simulink library "suspention"  (R2019b)
settings: Solver=ode45  StartTime=0.0  StopTime=10.0  RelTol=1e-3
PostLoadFcn:
  | setsysloc libsb2slobsolete
undefined symbols (not defined in the file): A, Ac, Ad, B, Bc, Bd, C, Cc, Cd, code, const, D, data, Dc, Dd, DiscIntNeverNeededParam, gain, info, k, m, map, no, stat, X0, xd, xi
libraries: $bdroot x2, simulink x2, libsb2sl x1
(part 2 of 2)

== system suspention/DYN/DResetIntegrator ==
  1stOrder : Subsystem  mask(DYN-Palette){IMODE=Forward Euler, RMODE=Single edge, K=1, X0=0, TS=0.1}
      mask prompts: IMODE "Integrator Method:"; RMODE "External Reset:"; K "Output Gains:"; X0 "Initial Conditions:"; TS "Sampling Time:"
      mask help: Nth order integration of an input with resettable states.
      mask init:
      | operator={'rising','either'};
      | method={'ForwardEuler';'BackwardEuler';'Trapezoidal'};
      | set_param([gcb  '/Integrator'],'ExternalReset',operator{RMODE},'IntegratorMethod',method{IMODE});
      | [x,y]=sblibico('1stOrderReset','disc');
      mask TypeOptions IMODE: Forward Euler | Backward Euler | Trapezoidal
      mask TypeOptions RMODE: Single edge | Double edge
      mask Display: plot(0,0,1,1,x,y)
  1stOrder1 : Subsystem  mask(DYN-Palette){IMODE=Forward Euler, RMODE=Single edge, X0=0, TS=0.1}
      mask prompts: IMODE "Integrator Method:"; RMODE "External Reset:"; X0 "Initial Conditions:"; TS "Sampling Time:"
      mask help: Nth order integration of an input with resettable states.
      mask init:
      | operator={'rising','either'};
      | method={'ForwardEuler';'BackwardEuler';'Trapezoidal'};
      | set_param([gcb  '/Integrator'],'ExternalReset',operator{RMODE},'IntegratorMethod',method{IMODE});
      | [x,y]=sblibico('1stOrder1Reset','disc');
      mask TypeOptions IMODE: Forward Euler | Backward Euler | Trapezoidal
      mask TypeOptions RMODE: Single edge | Double edge
      mask Display: plot(0,0,1,1,x,y)
  NthOrder : Subsystem  mask(DYN-Palette){IMODE=Forward Euler, N=1, RMODE=Single edge, NR=1, K=1, X0=0, TS=0.1}
      mask prompts: IMODE "Integrator Method:"; N "Order of Integration:"; RMODE "External Reset:"; NR "Highest Order of Resettable State:"; K "Output Gains:"; X0 "Initial Conditions:"; TS "Sampling Time:"
      mask help: Nth order integration of an input with resettable states.
      mask init:
      | no=length(K);
      | [stateMap,resetMap]=sblibdrv('Integrator',N,no,NR);
      | operator={'rising','either'};
      | method={'ForwardEuler';'BackwardEuler';'Trapezoidal'};
      | set_param([gcb  '/Integrator'],'ExternalReset',operator{RMODE},'IntegratorMethod',method{IMODE});
      | [x,y]=sblibico('nthOrderReset','disc');
      mask TypeOptions IMODE: Forward Euler | Backward Euler | Trapezoidal
      mask TypeOptions RMODE: Single edge | Double edge
      mask Display: plot(0,0,1,1,x,y)
  NthOrder1 : Subsystem  mask(DYN-Palette){IMODE=Forward Euler, N=1, RMODE=Single edge, NR=1, X0=0, TS=0.1}
      mask prompts: IMODE "Integrator Method:"; N "Order of Integration:"; RMODE "External Reset:"; NR "Highest Order of Resettable State:"; X0 "Initial Conditions:"; TS "Sampling Time:"
      mask help: Nth order integration of an input with resettable states.
      mask init:
      | no=length(X0)/N;
      | [stateMap,resetMap]=sblibdrv('Integrator',N,no,NR);
      | operator={'rising','either'};
      | method={'ForwardEuler';'BackwardEuler';'Trapezoidal'};
      | set_param([gcb  '/Integrator'],'ExternalReset',operator{RMODE},'IntegratorMethod',method{IMODE});
      | [x,y]=sblibico('nthOrder1Reset','disc');
      mask TypeOptions IMODE: Forward Euler | Backward Euler | Trapezoidal
      mask TypeOptions RMODE: Single edge | Double edge
      mask Display: plot(0,0,1,1,x,y)

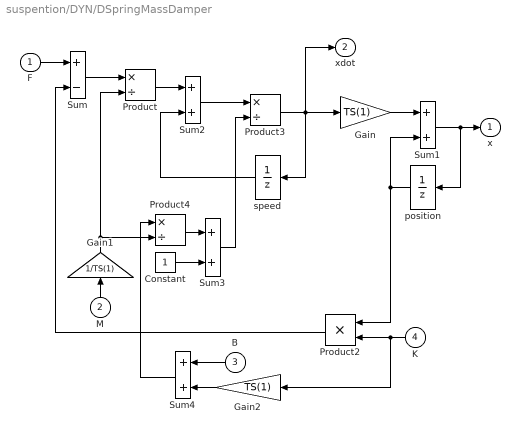
== system suspention/DYN/DSpringMassDamper ==
  F : Inport  SampleTime=TS
  M : Inport  Port=2  SampleTime=TS
  B : Inport  Port=3  SampleTime=TS
  K : Inport  Port=4  SampleTime=TS
  Constant : Constant
  Gain : Gain  Gain=TS(1)  SaturateOnIntegerOverflow=on  OutDataTypeStr=Inherit: Same as input  ParamDataTypeStr=Inherit: Same as input
  Gain1 : Gain  Gain=1/TS(1)  SaturateOnIntegerOverflow=on  OutDataTypeStr=Inherit: Same as input  ParamDataTypeStr=Inherit: Same as input
  Gain2 : Gain  Gain=TS(1)  SaturateOnIntegerOverflow=on  OutDataTypeStr=Inherit: Same as input  ParamDataTypeStr=Inherit: Same as input
  Product : Product  Inputs=*/  SaturateOnIntegerOverflow=on  RndMeth=Zero  InputSameDT=on  OutDataTypeStr=Inherit: Same as first input
  Product2 : Product  SaturateOnIntegerOverflow=on  RndMeth=Zero  InputSameDT=on  OutDataTypeStr=Inherit: Same as first input
  Product3 : Product  Inputs=*/  SaturateOnIntegerOverflow=on  RndMeth=Zero  InputSameDT=on  OutDataTypeStr=Inherit: Same as first input
  Product4 : Product  Inputs=*/  SaturateOnIntegerOverflow=on  RndMeth=Zero  InputSameDT=on  OutDataTypeStr=Inherit: Same as first input
  Sum : Sum  Inputs=+-  SaturateOnIntegerOverflow=on  InputSameDT=on  OutDataTypeStr=Inherit: Same as first input
  Sum{1..4} (4 alike) : Sum  SaturateOnIntegerOverflow=on  InputSameDT=on  OutDataTypeStr=Inherit: Same as first input
  position : UnitDelay  InitialCondition=X0(1)  SampleTime=TS  HasFrameUpgradeWarning=on
  speed : UnitDelay  InitialCondition=X0(2)  SampleTime=TS  HasFrameUpgradeWarning=on
  x : Outport  InitialOutput=X0(1)
  xdot : Outport  Port=2  InitialOutput=X0(2)
  wires:
  Sum4/1 -> Product4/1
  Gain2/1 -> Sum4/2
  B/1 -> Sum4/1
  K/1 -> Gain2/1, Product2/2
  Gain1/1 -> Product4/2, Product/2
  M/1 -> Gain1/1
  position/1 -> Product2/1, Sum1/2
  Sum3/1 -> Product3/2
  Product2/1 -> Sum/2
  Sum1/1 -> position/1, x/1
  Gain/1 -> Sum1/1
  Product3/1 -> xdot/1, Gain/1, speed/1
  Product4/1 -> Sum3/1
  Constant/1 -> Sum3/2
  speed/1 -> Sum2/2
  Sum2/1 -> Product3/1
  Product/1 -> Sum2/1
  Sum/1 -> Product/1
  F/1 -> Sum/1

== system suspention/DYN/DStateSpace ==
  u : Inport
  StateSpace : DiscreteStateSpace  A=A  B=B  C=C  D=D  InitialCondition=X0  SampleTime=TS
  y : Outport
  wires:
  u/1 -> StateSpace/1
  StateSpace/1 -> y/1

== system suspention/DYN/DTimeDelay ==
  u : Inport  SampleTime=TS
  Demux : Demux  Outputs=[no no (k+1)*no]
  Mux : Mux  Inputs=[no (k+1)*no]
  Selector : Selector  InputPortWidth=(k+2)*no  IndexOptions=Index vector (dialog)  Indices=[k*no+1:(k+2)*no 1:(k+1)*no]  OutputSizes=1
  Sum : Sum  Inputs=+|+  SaturateOnIntegerOverflow=on  InputSameDT=on  OutDataTypeStr=Inherit: Same as first input
  Unit Delay : UnitDelay  InitialCondition=X0  SampleTime=TS  HasFrameUpgradeWarning=on
  m : Gain  Gain=1-m  SaturateOnIntegerOverflow=on  OutDataTypeStr=Inherit: Same as input  ParamDataTypeStr=Inherit: Same as input
  m1 : Gain  Gain=m  SaturateOnIntegerOverflow=on  OutDataTypeStr=Inherit: Same as input  ParamDataTypeStr=Inherit: Same as input
  y : Outport
  wires:
  u/1 -> Mux/1
  Unit Delay/1 -> Mux/2
  Mux/1 -> Selector/1
  Sum/1 -> y/1
  m1/1 -> Sum/2
  m/1 -> Sum/1
  Demux/2 -> m1/1
  Demux/1 -> m/1
  Demux/3 -> Unit Delay/1
  Selector/1 -> Demux/1

== system suspention/LOG/Decoder ==
  u : Inport
  decoder : S-Function  FunctionName=sbdecoder  Parameters=BPI,MIN,MAX  SFunctionDeploymentMode=off  EnableBusSupport=off
  y : Outport
  wires:
  u/1 -> decoder/1
  decoder/1 -> y/1

== system suspention/LOG/EQV ==
  u1 : Inport
  u2 : Inport  Port=2
  EQV : Logic  Operator=NOT  Inputs=1
  NEQV : Logic  Operator=XOR
  bool1 : RelationalOperator  Operator=>  RndMeth=Nearest  InputSameDT=on
  bool2 : RelationalOperator  Operator=>  RndMeth=Nearest  InputSameDT=on
  zero : Constant  Value=0  OutDataTypeStr=Inherit: Inherit via back propagation
  y : Outport
  wires:
  bool1/1 -> NEQV/1
  bool2/1 -> NEQV/2
  u1/1 -> bool1/1
  u2/1 -> bool2/1
  zero/1 -> bool2/2, bool1/2
  NEQV/1 -> EQV/1
  EQV/1 -> y/1

== system suspention/LOG/Encoder ==
  u : Inport
  encoder : S-Function  FunctionName=sbencoder  Parameters=BPO,MIN,MAX  SFunctionDeploymentMode=off  EnableBusSupport=off
  y : Outport
  wires:
  u/1 -> encoder/1
  encoder/1 -> y/1

== system suspention/LOG/GainScheduler ==
  s : Inport
  u : Inport  Port=2
  sbgainsched : S-Function  FunctionName=sbgainsched  Parameters=IND,GAIN  SFunctionDeploymentMode=off  EnableBusSupport=off
  y : Outport
  wires:
  s/1 -> sbgainsched/1
  sbgainsched/1 -> y/1
  u/1 -> sbgainsched/2

== system suspention/LOG/LogExpression ==
  u : Inport
  sblogexp : S-Function  FunctionName=sblogexp  Parameters=code,stat,data,info,P0,TS  SFunctionDeploymentMode=off  EnableBusSupport=off
  y : Outport
  wires:
  u/1 -> sblogexp/1
  sblogexp/1 -> y/1

== system suspention/LOG/NEQV ==
  u1 : Inport
  u2 : Inport  Port=2
  NEQV : Logic  Operator=XOR
  bool1 : RelationalOperator  Operator=>  RndMeth=Nearest  InputSameDT=on
  bool2 : RelationalOperator  Operator=>  RndMeth=Nearest  InputSameDT=on
  zero : Constant  Value=0  OutDataTypeStr=Inherit: Inherit via back propagation
  y : Outport
  wires:
  bool1/1 -> NEQV/1
  bool2/1 -> NEQV/2
  u1/1 -> bool1/1
  NEQV/1 -> y/1
  u2/1 -> bool2/1
  zero/1 -> bool1/2, bool2/2

== system suspention/LOG/NOT ==
  u1 : Inport
  bool1 : RelationalOperator  Operator=>  RndMeth=Nearest  InputSameDT=on
  logic : Logic  Operator=NOT
  zero : Constant  Value=0  OutDataTypeStr=Inherit: Inherit via back propagation
  y : Outport
  wires:
  bool1/1 -> logic/1
  u1/1 -> bool1/1
  logic/1 -> y/1
  zero/1 -> bool1/2

== system suspention/LOG/ShiftRegister ==
  u : Inport  SampleTime=TS
  sbshiftreg : S-Function  FunctionName=sbshiftreg  Parameters=NX,NY,X0,TS  SFunctionDeploymentMode=off  EnableBusSupport=off
  y : Outport
  wires:
  u/1 -> sbshiftreg/1
  sbshiftreg/1 -> y/1

== system suspention/LOG/Switch ==
  u1 : Inport
  u2 : Inport  Port=2
  u3 : Inport  Port=3
  Switch : Switch  Criteria=u2 > Threshold  SaturateOnIntegerOverflow=on  InputSameDT=on
  y : Outport
  wires:
  Switch/1 -> y/1
  u2/1 -> Switch/1
  u3/1 -> Switch/3
  u1/1 -> Switch/2

== system suspention/MAT/Constant ==
  Constant : Constant  Value=constantValue
  Y : Outport
  wires:
  Constant/1 -> Y/1

== system suspention/MAT/LeftMultiply ==
  A : Inport
  Matrix Gain : Gain  Gain=G  Multiplication=Matrix(u*K)  SaturateOnIntegerOverflow=on  OutDataTypeStr=Inherit: Same as input  ParamDataTypeStr=Inherit: Same as input
  Y2y : Reshape
  a2A : Reshape  OutputDimensionality=Customize  OutputDimensions=[nACols,nARows]
  Y : Outport
  wires:
  A/1 -> a2A/1
  Y2y/1 -> Y/1
  Matrix Gain/1 -> Y2y/1
  a2A/1 -> Matrix Gain/1

== system suspention/MAT/MatLeftDivide ==
  A : Inport
  B : Inport  Port=2
  Product : Product  Inputs=*/  Multiplication=Matrix(*)  SaturateOnIntegerOverflow=on  RndMeth=Zero  InputSameDT=on  OutDataTypeStr=Inherit: Same as first input
  Y2y : Reshape
  a2A : Reshape  OutputDimensionality=Customize  OutputDimensions=[nACols,nARows]
  b2B : Reshape  OutputDimensionality=Customize  OutputDimensions=[nBCols,nBRows]
  Y : Outport
  wires:
  Product/1 -> Y2y/1
  B/1 -> b2B/1
  Y2y/1 -> Y/1
  A/1 -> a2A/1
  b2B/1 -> Product/1
  a2A/1 -> Product/2

== system suspention/MAT/MatRightDivide ==
  A : Inport
  B : Inport  Port=2
  Product : Product  Inputs=/*  Multiplication=Matrix(*)  SaturateOnIntegerOverflow=on  RndMeth=Zero  InputSameDT=on  OutDataTypeStr=Inherit: Same as first input
  Y2y : Reshape
  a2A : Reshape  OutputDimensionality=Customize  OutputDimensions=[nACols,nARows]
  b2B : Reshape  OutputDimensionality=Customize  OutputDimensions=[nBCols,nBRows]
  Y : Outport
  wires:
  b2B/1 -> Product/2
  a2A/1 -> Product/1
  Product/1 -> Y2y/1
  A/1 -> a2A/1
  Y2y/1 -> Y/1
  B/1 -> b2B/1

== system suspention/MAT/MatrixInverse ==
  A : Inport
  Product : Product  Inputs=/  Multiplication=Matrix(*)  SaturateOnIntegerOverflow=on  RndMeth=Zero  InputSameDT=on  OutDataTypeStr=Inherit: Same as first input
  Y2y : Reshape
  a2A : Reshape  OutputDimensionality=Customize  OutputDimensions=[nACols,nARows]
  Y : Outport
  wires:
  A/1 -> a2A/1
  Y2y/1 -> Y/1
  a2A/1 -> Product/1
  Product/1 -> Y2y/1

== system suspention/MAT/MatrixMultiply ==
  A : Inport
  B : Inport  Port=2
  Product : Product  Inputs=**  Multiplication=Matrix(*)  SaturateOnIntegerOverflow=on  RndMeth=Zero  InputSameDT=on  OutDataTypeStr=Inherit: Same as first input
  Y2y : Reshape
  a2A : Reshape  OutputDimensionality=Customize  OutputDimensions=[nACols,nARows]
  b2B : Reshape  OutputDimensionality=Customize  OutputDimensions=[nBCols,nBRows]
  Y : Outport
  wires:
  a2A/1 -> Product/2
  b2B/1 -> Product/1
  B/1 -> b2B/1
  Y2y/1 -> Y/1
  A/1 -> a2A/1
  Product/1 -> Y2y/1

== system suspention/MAT/MatrixTranspose ==
  A : Inport
  Selector : Selector  InputPortWidth=nARows*nACols  IndexOptions=Index vector (dialog)  Indices=mapIndices(:)  OutputSizes=1
  Y : Outport
  wires:
  Selector/1 -> Y/1
  A/1 -> Selector/1

== system suspention/MAT/RightMultiply ==
  A : Inport
  Matrix Gain : Gain  Gain=G  Multiplication=Matrix(K*u)  SaturateOnIntegerOverflow=on  OutDataTypeStr=Inherit: Same as input  ParamDataTypeStr=Inherit: Same as input
  Y2y : Reshape
  a2A : Reshape  OutputDimensionality=Customize  OutputDimensions=[nACols,nARows]
  Y : Outport
  wires:
  a2A/1 -> Matrix Gain/1
  Matrix Gain/1 -> Y2y/1
  Y2y/1 -> Y/1
  A/1 -> a2A/1

== system suspention/NTP/BiCubicInterp ==
  note: Swap inputs to accommodate
      | Row-major 2-D tables in
      | SystemBuild
  u1 : Inport
  u2 : Inport  Port=2
  Look-Up Table (n-D) : Lookup_n-D  BreakpointsForDimension1=in2BrkPoints  BreakpointsForDimension2=in1BrkPoints  BeginIndexSearchUsingPreviousIndexResult=on  Table=outBrkPoints  InterpMethod=Cubic spline  ExtrapMethod=Clip  DiagnosticForOutOfRangeInput=Error  RndMeth=Simplest  InputSameDT=on
  y : Outport
  wires:
  u1/1 -> Look-Up Table (n-D)/2
  u2/1 -> Look-Up Table (n-D)/1
  Look-Up Table (n-D)/1 -> y/1

== system suspention/NTP/BiLinearInterp ==
  note: Swap inputs to accommodate
      | Row-major 2-D tables in
      | SystemBuild
  u1 : Inport
  u2 : Inport  Port=2
  Look-Up Table (n-D) : Lookup_n-D  BreakpointsForDimension1=in2BrkPoints  BreakpointsForDimension2=in1BrkPoints  BeginIndexSearchUsingPreviousIndexResult=on  Table=outBrkPoints  RndMeth=Simplest  InputSameDT=on
  y : Outport
  wires:
  u2/1 -> Look-Up Table (n-D)/1
  u1/1 -> Look-Up Table (n-D)/2
  Look-Up Table (n-D)/1 -> y/1

== system suspention/NTP/ConstantInterp ==
  u : Inport
  Look-Up Table (n-D) : Lookup_n-D  NumberOfTableDimensions=1  BreakpointsForDimension1=in1BrkPoints  BreakpointsForDimension2=[1:3]  BeginIndexSearchUsingPreviousIndexResult=on  UseOneInputPortForAllInputData=on  Table=outBrkPoints  InterpMethod=Flat  ExtrapMethod=Clip  RndMeth=Simplest  InputSameDT=on
  y : Outport
  wires:
  Look-Up Table (n-D)/1 -> y/1
  u/1 -> Look-Up Table (n-D)/1

== system suspention/NTP/CubicInterp ==
  u : Inport
  Look-Up Table (n-D) : Lookup_n-D  NumberOfTableDimensions=1  BreakpointsForDimension1=in1BrkPoints  BreakpointsForDimension2=[1:3]  BeginIndexSearchUsingPreviousIndexResult=on  UseOneInputPortForAllInputData=on  Table=outBrkPoints  InterpMethod=Cubic spline  ExtrapMethod=Cubic spline  RndMeth=Simplest  InputSameDT=on
  y : Outport
  wires:
  u/1 -> Look-Up Table (n-D)/1
  Look-Up Table (n-D)/1 -> y/1

== system suspention/NTP/LinearInterp ==
  u : Inport
  Look-Up Table (n-D) : Lookup_n-D  NumberOfTableDimensions=1  BreakpointsForDimension1=in1BrkPoints  BreakpointsForDimension2=[1:3]  BeginIndexSearchUsingPreviousIndexResult=on  UseOneInputPortForAllInputData=on  Table=outBrkPoints  RndMeth=Simplest  InputSameDT=on
  y : Outport
  wires:
  u/1 -> Look-Up Table (n-D)/1
  Look-Up Table (n-D)/1 -> y/1

== system suspention/NTP/MultiLinearInterp ==
  u : Inport
  multilinear interp : Lookup_n-D  NumberOfTableDimensions=NINP+1  BreakpointsForDimension1=in1BrkPoints  BreakpointsForDimension2=in2BrkPoints  BreakpointsForDimension3=in3BrkPoints  BreakpointsForDimension4=in4BrkPoints  BreakpointsForDimension5=in5BrkPoints  BreakpointsForDimension6=in6BrkPoints  BreakpointsForDimension7=in7BrkPoints  BreakpointsForDimension8=in8BrkPoints  IndexSearchMethod=Linear search  BeginIndexSearchUsingPreviousIndexResult=on  UseOneInputPortForAllInputData=on  Table=tableData  RndMeth=Simplest  InputSameDT=on
  y : Outport
  wires:
  multilinear interp/1 -> y/1
  u/1 -> multilinear interp/1

== system suspention/PEL/Constant**u ==
  u : Inport
  Constant : Constant  Value=CONST
  Power : Math  Operator=pow  SaturateOnIntegerOverflow=on
  y : Outport
  wires:
  Power/1 -> y/1
  Constant/1 -> Power/1
  u/1 -> Power/2

== system suspention/PEL/SignedSqrt ==
  u : Inport
  Abs : Abs  SaturateOnIntegerOverflow=on
  Math Function : Math  Operator=sqrt  SaturateOnIntegerOverflow=on
  Product : Product  SaturateOnIntegerOverflow=on  RndMeth=Zero  InputSameDT=on  OutDataTypeStr=Inherit: Same as first input
  Sign : Signum
  y : Outport
  wires:
  Math Function/1 -> Product/1
  Sign/1 -> Product/2
  Abs/1 -> Math Function/1
  Product/1 -> y/1
  u/1 -> Abs/1, Sign/1

== system suspention/PEL/u**Constant ==
  u : Inport
  Constant : Constant  Value=CONST
  Power : Math  Operator=pow  SaturateOnIntegerOverflow=on
  y : Outport
  wires:
  Power/1 -> y/1
  u/1 -> Power/1
  Constant/1 -> Power/2

== system suspention/PWL/Preload ==
  u : Inport
  Constant : Constant  Value=preload
  Constant1 : Constant  Value=-preload
  Sum : Sum  SaturateOnIntegerOverflow=on  InputSameDT=on  OutDataTypeStr=Inherit: Same as first input
  Switch : Switch  SaturateOnIntegerOverflow=on  InputSameDT=on
  slope : Gain  Gain=slope  SaturateOnIntegerOverflow=on  OutDataTypeStr=Inherit: Same as input  ParamDataTypeStr=Inherit: Same as input
  y : Outport
  wires:
  slope/1 -> Sum/2
  Switch/1 -> Sum/1
  u/1 -> Switch/2, slope/1
  Sum/1 -> y/1
  Constant/1 -> Switch/1
  Constant1/1 -> Switch/3

== system suspention/PWL/Quantization ==
  u : Inport
  Resolution : Constant  Value=RES
  Type : Rounding  Operator=round
  div : Product  Inputs=*/  SaturateOnIntegerOverflow=on  RndMeth=Zero  InputSameDT=on  OutDataTypeStr=Inherit: Same as first input
  mul : Product  SaturateOnIntegerOverflow=on  RndMeth=Zero  InputSameDT=on  OutDataTypeStr=Inherit: Same as first input
  y : Outport
  wires:
  div/1 -> Type/1
  Type/1 -> mul/1
  Resolution/1 -> div/2, mul/2
  u/1 -> div/1
  mul/1 -> y/1

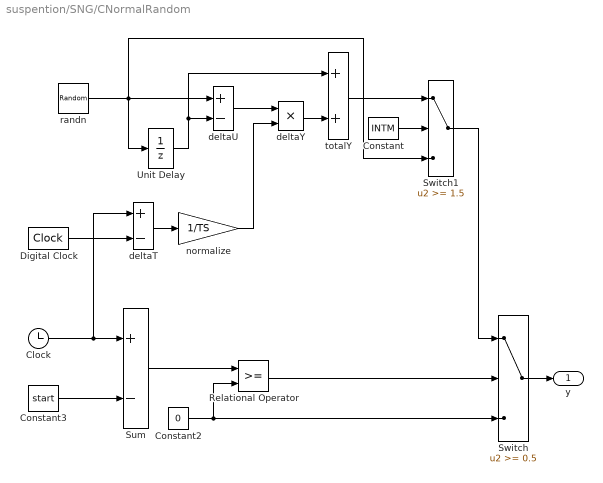
== system suspention/SNG/CNormalRandom ==
  Clock : Clock
  Constant : Constant  Value=INTM
  Constant2 : Constant  Value=0
  Constant3 : Constant  Value=start
  Digital Clock : DigitalClock  SampleTime=TS
  Relational Operator : RelationalOperator  RndMeth=Nearest  InputSameDT=on
  Sum : Sum  Inputs=+-  SaturateOnIntegerOverflow=on  InputSameDT=on  OutDataTypeStr=Inherit: Same as first input
  Switch : Switch  Threshold=0.5  SaturateOnIntegerOverflow=on  InputSameDT=on
  Switch1 : Switch  Threshold=1.5  SaturateOnIntegerOverflow=on  InputSameDT=on
  Unit Delay : UnitDelay  SampleTime=TS  HasFrameUpgradeWarning=on
  deltaT : Sum  Inputs=+-  SaturateOnIntegerOverflow=on  InputSameDT=on  OutDataTypeStr=Inherit: Same as first input
  deltaU : Sum  Inputs=+-  SaturateOnIntegerOverflow=on  InputSameDT=on  OutDataTypeStr=Inherit: Same as first input
  deltaY : Product  SaturateOnIntegerOverflow=on  RndMeth=Zero  InputSameDT=on  OutDataTypeStr=Inherit: Same as first input
  normalize : Gain  Gain=1/TS  SaturateOnIntegerOverflow=on  OutDataTypeStr=Inherit: Same as input  ParamDataTypeStr=Inherit: Same as input
  randn : RandomNumber  Mean=MEAN  Variance=STD.^2  Seed=SEED  SampleTime=TS
  totalY : Sum  SaturateOnIntegerOverflow=on  InputSameDT=on  OutDataTypeStr=Inherit: Same as first input
  y : Outport
  wires:
  Clock/1 -> deltaT/1, Sum/1
  Switch/1 -> y/1
  Switch1/1 -> Switch/1
  Constant2/1 -> Switch/3, Relational Operator/2
  Relational Operator/1 -> Switch/2
  Sum/1 -> Relational Operator/1
  Constant3/1 -> Sum/2
  randn/1 -> deltaU/1, Unit Delay/1, Switch1/3
  Constant/1 -> Switch1/2
  totalY/1 -> Switch1/1
  Unit Delay/1 -> deltaU/2, totalY/1
  deltaY/1 -> totalY/2
  normalize/1 -> deltaY/2
  deltaU/1 -> deltaY/1
  deltaT/1 -> normalize/1
  Digital Clock/1 -> deltaT/2

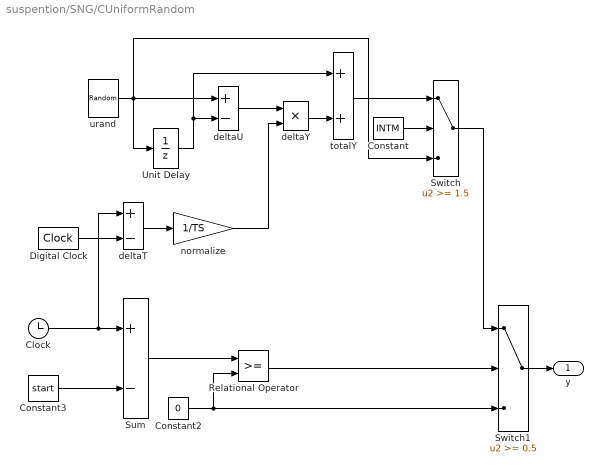
== system suspention/SNG/CUniformRandom ==
  Clock : Clock
  Constant : Constant  Value=INTM
  Constant2 : Constant  Value=0
  Constant3 : Constant  Value=start
  Digital Clock : DigitalClock  SampleTime=TS
  Relational Operator : RelationalOperator  RndMeth=Nearest  InputSameDT=on
  Sum : Sum  Inputs=+-  SaturateOnIntegerOverflow=on  InputSameDT=on  OutDataTypeStr=Inherit: Same as first input
  Switch : Switch  Threshold=1.5  SaturateOnIntegerOverflow=on  InputSameDT=on
  Switch1 : Switch  Threshold=0.5  SaturateOnIntegerOverflow=on  InputSameDT=on
  Unit Delay : UnitDelay  SampleTime=TS  HasFrameUpgradeWarning=on
  deltaT : Sum  Inputs=+-  SaturateOnIntegerOverflow=on  InputSameDT=on  OutDataTypeStr=Inherit: Same as first input
  deltaU : Sum  Inputs=+-  SaturateOnIntegerOverflow=on  InputSameDT=on  OutDataTypeStr=Inherit: Same as first input
  deltaY : Product  SaturateOnIntegerOverflow=on  RndMeth=Zero  InputSameDT=on  OutDataTypeStr=Inherit: Same as first input
  normalize : Gain  Gain=1/TS  SaturateOnIntegerOverflow=on  OutDataTypeStr=Inherit: Same as input  ParamDataTypeStr=Inherit: Same as input
  totalY : Sum  SaturateOnIntegerOverflow=on  InputSameDT=on  OutDataTypeStr=Inherit: Same as first input
  urand : UniformRandomNumber  Minimum=MIN  Maximum=MAX  Seed=SEED  SampleTime=TS
  y : Outport
  wires:
  Constant2/1 -> Relational Operator/2, Switch1/3
  Relational Operator/1 -> Switch1/2
  Sum/1 -> Relational Operator/1
  Constant3/1 -> Sum/2
  Switch1/1 -> y/1
  Constant/1 -> Switch/2
  totalY/1 -> Switch/1
  Unit Delay/1 -> totalY/1, deltaU/2
  deltaY/1 -> totalY/2
  normalize/1 -> deltaY/2
  deltaU/1 -> deltaY/1
  deltaT/1 -> normalize/1
  Digital Clock/1 -> deltaT/2
  urand/1 -> Switch/3, Unit Delay/1, deltaU/1
  Switch/1 -> Switch1/1
  Clock/1 -> Sum/1, deltaT/1

== system suspention/SNG/DNormalRandom ==
  Clock : Clock
  Constant2 : Constant  Value=0
  Constant3 : Constant  Value=start
  Relational Operator : RelationalOperator  RndMeth=Nearest  InputSameDT=on
  Sum : Sum  Inputs=+-  SaturateOnIntegerOverflow=on  InputSameDT=on  OutDataTypeStr=Inherit: Same as first input
  Switch : Switch  Threshold=0.5  SaturateOnIntegerOverflow=on  InputSameDT=on
  randn : RandomNumber  Mean=MEAN  Variance=STD.^2  Seed=SEED  SampleTime=TS
  y : Outport
  wires:
  randn/1 -> Switch/1
  Clock/1 -> Sum/1
  Constant3/1 -> Sum/2
  Sum/1 -> Relational Operator/1
  Relational Operator/1 -> Switch/2
  Constant2/1 -> Relational Operator/2, Switch/3
  Switch/1 -> y/1

== system suspention/SNG/DUniformRandom ==
  Clock : Clock
  Constant2 : Constant  Value=0
  Constant3 : Constant  Value=start
  Relational Operator : RelationalOperator  RndMeth=Nearest  InputSameDT=on
  Sum : Sum  Inputs=+-  SaturateOnIntegerOverflow=on  InputSameDT=on  OutDataTypeStr=Inherit: Same as first input
  Switch : Switch  Threshold=0.5  SaturateOnIntegerOverflow=on  InputSameDT=on
  urand : UniformRandomNumber  Minimum=MIN  Maximum=MAX  Seed=SEED  SampleTime=TS
  y : Outport
  wires:
  Clock/1 -> Sum/1
  Constant3/1 -> Sum/2
  Sum/1 -> Relational Operator/1
  Relational Operator/1 -> Switch/2
  Constant2/1 -> Switch/3, Relational Operator/2
  Switch/1 -> y/1
  urand/1 -> Switch/1

== system suspention/SNG/GenWaveform ==
  Clock : Clock
  Constant1 : Constant  Value=period
  Constant2 : Constant  Value=0
  Constant3 : Constant  Value=start
  LinearInterp : libsb2sl/NTP/LinearInterp  in1BrkPoints=in1BrkPoints  outBrkPoints=outBrkPoints
      settings: SourceProductName=Simulink  SourceProductBaseCode=SL
  Math Function : Math  Operator=rem  SaturateOnIntegerOverflow=on
  Sum : Sum  Inputs=+-  SaturateOnIntegerOverflow=on  InputSameDT=on  OutDataTypeStr=Inherit: Same as first input
  Switch : Switch  SaturateOnIntegerOverflow=on  InputSameDT=on
  y : Outport
  wires:
  Clock/1 -> Sum/1
  Switch/1 -> y/1
  Sum/1 -> Math Function/1, Switch/2
  Constant3/1 -> Sum/2
  Constant2/1 -> Switch/3
  Constant1/1 -> Math Function/2
  Math Function/1 -> LinearInterp/1
  LinearInterp/1 -> Switch/1

== system suspention/SNG/LimRamp ==
  Compare To Zero : simulink/Logic and Bit Operations/Compare To Zero  relop=~=  OutDataTypeStr=boolean  ZeroCross=off
  Constant5 : Constant  Value=SAT
  Constant6 : Constant  Value=RATE
  Data Type Conversion : DataTypeConversion
  Product : Product  SaturateOnIntegerOverflow=on  RndMeth=Zero  InputSameDT=on  OutDataTypeStr=Inherit: Same as first input
  Product1 : Product  SaturateOnIntegerOverflow=on  RndMeth=Zero  InputSameDT=on  OutDataTypeStr=Inherit: Same as first input
  Ramp : simulink/Sources/Ramp  slope=RATE  start=start  InitialOutput=0
  Sum1 : Sum  Inputs=-+  SaturateOnIntegerOverflow=on  InputSameDT=on  OutDataTypeStr=Inherit: Same as first input
  Switch1 : Switch  SaturateOnIntegerOverflow=on  InputSameDT=on
  y : Outport
  wires:
  Data Type Conversion/1 -> Product1/2
  Product1/1 -> Switch1/3
  Compare To Zero/1 -> Data Type Conversion/1
  Ramp/1 -> Compare To Zero/1, Switch1/1, Sum1/1
  Constant6/1 -> Product/2
  Sum1/1 -> Product/1
  Constant5/1 -> Product1/1, Sum1/2
  Switch1/1 -> y/1
  Product/1 -> Switch1/2

== system suspention/SNG/PulseTrain ==
  Pulse Generator1 : DiscretePulseGenerator  PulseType=Time based  Amplitude=A  Period=1./F  PulseWidth=PW.*F*100  PhaseDelay=start
  y : Outport
  wires:
  Pulse Generator1/1 -> y/1

== system suspention/SNG/SinusoidGen ==
  Clock : Clock
  Constant2 : Constant  Value=0
  Constant3 : Constant  Value=start
  Relational Operator : RelationalOperator  RndMeth=Nearest  InputSameDT=on
  Sine Wave : Sin  TimeSource=Use external signal  Amplitude=A  Frequency=2*pi*F  Phase=pi*PHI/180  SampleTime=0
  Sum : Sum  Inputs=+-  SaturateOnIntegerOverflow=on  InputSameDT=on  OutDataTypeStr=Inherit: Same as first input
  Switch : Switch  Threshold=0.5  SaturateOnIntegerOverflow=on  InputSameDT=on
  y : Outport
  wires:
  Switch/1 -> y/1
  Sine Wave/1 -> Switch/1
  Constant2/1 -> Switch/3, Relational Operator/2
  Relational Operator/1 -> Switch/2
  Constant3/1 -> Sum/2
  Clock/1 -> Sum/1
  Sum/1 -> Sine Wave/1, Relational Operator/1

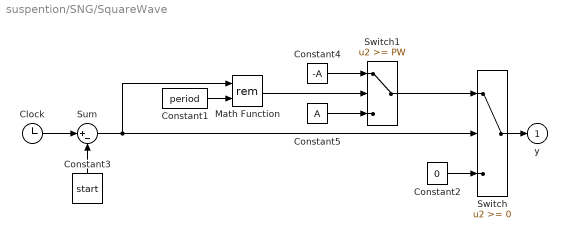
== system suspention/SNG/SquareWave ==
  Clock : Clock
  Constant1 : Constant  Value=period
  Constant2 : Constant  Value=0
  Constant3 : Constant  Value=start
  Constant4 : Constant  Value=-A
  Constant5 : Constant  Value=A
  Math Function : Math  Operator=rem  SaturateOnIntegerOverflow=on
  Sum : Sum  Inputs=|+-  SaturateOnIntegerOverflow=on  InputSameDT=on  OutDataTypeStr=Inherit: Same as first input
  Switch : Switch  SaturateOnIntegerOverflow=on  InputSameDT=on
  Switch1 : Switch  Threshold=PW  SaturateOnIntegerOverflow=on  InputSameDT=on
  y : Outport
  wires:
  Constant5/1 -> Switch1/3
  Constant4/1 -> Switch1/1
  Switch1/1 -> Switch/1
  Math Function/1 -> Switch1/2
  Switch/1 -> y/1
  Constant3/1 -> Sum/2
  Sum/1 -> Math Function/1, Switch/2
  Clock/1 -> Sum/1
  Constant2/1 -> Switch/3
  Constant1/1 -> Math Function/2

== system suspention/SNG/StepFcn ==
  Step : Step  Time=start  After=A  SampleTime=TS
  y : Outport
  wires:
  Step/1 -> y/1

== system suspention/SUP/DataStoreRW ==
  u : Inport  PortDimensions=NREG  SampleTime=TS
  Mux : Mux  Inputs=2
  Selector : Selector  InputPortWidth=inpWidth  IndexOptions=Index vector (dialog)  Indices=inputMap  OutputSizes=1
  dsRead : DataStoreRead  Priority=1  DataStoreName=VAR  SampleTime=TS
  dsWrite : DataStoreWrite  Priority=2  DataStoreName=VAR  SampleTime=TS
  y : Outport
  wires:
  u/1 -> Mux/1
  Mux/1 -> Selector/1
  dsRead/1 -> Mux/2
  Selector/1 -> dsWrite/1, y/1

== system suspention/SUP/DataStoreW ==
  u : Inport  PortDimensions=NREG  SampleTime=TS
  Mux : Mux  Inputs=2
  Selector : Selector  InputPortWidth=inpWidth  IndexOptions=Index vector (dialog)  Indices=inputMap  OutputSizes=1
  dsRead : DataStoreRead  Priority=1  DataStoreName=VAR  SampleTime=TS
  dsWrite : DataStoreWrite  Priority=2  DataStoreName=VAR  SampleTime=TS
  wires:
  Mux/1 -> Selector/1
  u/1 -> Mux/1
  Selector/1 -> dsWrite/1
  dsRead/1 -> Mux/2

== system suspention/TRG/CosAsin ==
  u : Inport
  Bias : Bias  Bias=1
  Gain : Gain  Gain=-1
  Product : Product  RndMeth=Zero
  Sqrt : Sqrt  SaturateOnIntegerOverflow=on
  y : Outport
  wires:
  u/1 -> Product/1, Product/2
  Product/1 -> Gain/1
  Bias/1 -> Sqrt/1
  Sqrt/1 -> y/1
  Gain/1 -> Bias/1

== system suspention/TRG/CosAtan2 ==
  u1 : Inport
  u2 : Inport  Port=2
  Add : Sum
  Divide : Product  Inputs=*/
  Product : Product  RndMeth=Zero
  Product1 : Product  RndMeth=Zero
  Sqrt : Sqrt  SaturateOnIntegerOverflow=on
  y : Outport
  wires:
  u1/1 -> Product/2, Product/1
  Product1/1 -> Add/2
  Add/1 -> Sqrt/1
  Product/1 -> Add/1
  u2/1 -> Product1/1, Divide/1, Product1/2
  Sqrt/1 -> Divide/2
  Divide/1 -> y/1

== system suspention/TRG/SinAtan2 ==
  u1 : Inport
  u2 : Inport  Port=2
  Add : Sum
  Divide : Product  Inputs=*/
  Product : Product  RndMeth=Zero
  Product1 : Product  RndMeth=Zero
  Sqrt : Sqrt  SaturateOnIntegerOverflow=on
  y : Outport
  wires:
  u1/1 -> Divide/1, Product/2, Product/1
  Product1/1 -> Add/2
  Add/1 -> Sqrt/1
  Product/1 -> Add/1
  u2/1 -> Product1/2, Product1/1
  Sqrt/1 -> Divide/2
  Divide/1 -> y/1

== system suspention/USR/BlockScript ==
  u : Inport
  BlockScriptCode : S-Function  FunctionName=foo  Parameters=SIZES,X0  SFunctionDeploymentMode=off  EnableBusSupport=off
  y : Outport
  wires:
  BlockScriptCode/1 -> y/1
  u/1 -> BlockScriptCode/1

== system suspention/USR/ZIBlockScript ==
  BlockScriptCode : S-Function  FunctionName=foo  Parameters=SIZES,X0  SFunctionDeploymentMode=off  EnableBusSupport=off
  Ground : Ground
  y : Outport
  wires:
  BlockScriptCode/1 -> y/1
  Ground/1 -> BlockScriptCode/1

== system suspention/ALG/AlgExpression/Constant ==
  Constant : Constant  Value=const
  y : Outport
  wires:
  Constant/1 -> y/1

== system suspention/ALG/AlgExpression/Offset ==
  u : Inport
  Constant : Constant  Value=const
  Gain : Gain  Gain=sign  SaturateOnIntegerOverflow=on  OutDataTypeStr=Inherit: Same as input  ParamDataTypeStr=Inherit: Same as input
  Selector : Selector  InputPortWidth=ni  IndexOptions=Index vector (dialog)  Indices=map  OutputSizes=1
  Sum : Sum  Inputs=|++  SaturateOnIntegerOverflow=on  InputSameDT=on  OutDataTypeStr=Inherit: Same as first input
  y : Outport
  wires:
  Constant/1 -> Sum/1
  Gain/1 -> Sum/2
  Sum/1 -> y/1
  Selector/1 -> Gain/1
  u/1 -> Selector/1

== system suspention/ALG/AlgExpression/PowerCU ==
  u : Inport
  Constant : Constant  Value=const
  Gain : Gain  Gain=sign  SaturateOnIntegerOverflow=on  OutDataTypeStr=Inherit: Same as input  ParamDataTypeStr=Inherit: Same as input
  Math Function : Math  Operator=pow  SaturateOnIntegerOverflow=on
  Selector : Selector  InputPortWidth=ni  IndexOptions=Index vector (dialog)  Indices=map  OutputSizes=1
  y : Outport
  wires:
  Math Function/1 -> Gain/1
  Gain/1 -> y/1
  Constant/1 -> Math Function/1
  u/1 -> Selector/1
  Selector/1 -> Math Function/2

== system suspention/ALG/AlgExpression/Product ==
  u : Inport
  Gain : Gain  Gain=sign  SaturateOnIntegerOverflow=on  OutDataTypeStr=Inherit: Same as input  ParamDataTypeStr=Inherit: Same as input
  Product : Product  Inputs=**  SaturateOnIntegerOverflow=on  RndMeth=Zero  InputSameDT=on  OutDataTypeStr=Inherit: Same as first input
  Selector : Selector  InputPortWidth=ni  IndexOptions=Index vector (dialog)  Indices=map(:,1)  OutputSizes=1
  Selector1 : Selector  InputPortWidth=ni  IndexOptions=Index vector (dialog)  Indices=map(:,2)  OutputSizes=1
  y : Outport
  wires:
  Gain/1 -> y/1
  Product/1 -> Gain/1
  u/1 -> Selector/1, Selector1/1
  Selector/1 -> Product/1
  Selector1/1 -> Product/2

== system suspention/ALG/AlgExpression/Reciprocal ==
  u : Inport
  Constant : Constant  Value=const
  Div : Product  Inputs=*/  SaturateOnIntegerOverflow=on  RndMeth=Zero  InputSameDT=on  OutDataTypeStr=Inherit: Same as first input
  Selector : Selector  InputPortWidth=ni  IndexOptions=Index vector (dialog)  Indices=map  OutputSizes=1
  y : Outport
  wires:
  u/1 -> Selector/1
  Selector/1 -> Div/2
  Constant/1 -> Div/1
  Div/1 -> y/1

== system suspention/ALG/AlgExpression/Scale ==
  u : Inport
  Gain : Gain  Gain=gain  SaturateOnIntegerOverflow=on  OutDataTypeStr=Inherit: Same as input  ParamDataTypeStr=Inherit: Same as input
  Selector : Selector  InputPortWidth=ni  IndexOptions=Index vector (dialog)  Indices=map  OutputSizes=1
  y : Outport
  wires:
  Gain/1 -> y/1
  Selector/1 -> Gain/1
  u/1 -> Selector/1

== system suspention/ALG/AlgExpression/Summation ==
  u : Inport
  Gain : Gain  Gain=sign(:,1)  SaturateOnIntegerOverflow=on  OutDataTypeStr=Inherit: Same as input  ParamDataTypeStr=Inherit: Same as input
  Gain1 : Gain  Gain=sign(:,2)  SaturateOnIntegerOverflow=on  OutDataTypeStr=Inherit: Same as input  ParamDataTypeStr=Inherit: Same as input
  Selector : Selector  InputPortWidth=ni  IndexOptions=Index vector (dialog)  Indices=map(:,1)  OutputSizes=1
  Selector1 : Selector  InputPortWidth=ni  IndexOptions=Index vector (dialog)  Indices=map(:,2)  OutputSizes=1
  Sum : Sum  Inputs=|++  SaturateOnIntegerOverflow=on  InputSameDT=on  OutDataTypeStr=Inherit: Same as first input
  y : Outport
  wires:
  Sum/1 -> y/1
  u/1 -> Selector1/1, Selector/1
  Gain1/1 -> Sum/2
  Selector1/1 -> Gain1/1
  Gain/1 -> Sum/1
  Selector/1 -> Gain/1

== system suspention/DYN/CIntegrator/1stOrder ==
  u : Inport
  Gain : Gain  Gain=K  SaturateOnIntegerOverflow=on  OutDataTypeStr=Inherit: Same as input  ParamDataTypeStr=Inherit: Same as input
  Integrator : Integrator  InitialCondition=X0
  y : Outport
  wires:
  Gain/1 -> y/1
  u/1 -> Integrator/1
  Integrator/1 -> Gain/1

== system suspention/DYN/CIntegrator/NthOrder ==
  u : Inport
  Demux : Demux  Outputs=[no no*N]
  Gain : Gain  Gain=K  SaturateOnIntegerOverflow=on  OutDataTypeStr=Inherit: Same as input  ParamDataTypeStr=Inherit: Same as input
  Integrator : Integrator  InitialCondition=X0
  Mux : Mux  Inputs=[no no*N]
  StateMap : Selector  InputPortWidth=no*(1+N)  IndexOptions=Index vector (dialog)  Indices=stateMap  OutputSizes=1
  y : Outport
  wires:
  Gain/1 -> y/1
  Demux/1 -> Gain/1
  u/1 -> Mux/1
  Demux/2 -> Integrator/1
  Integrator/1 -> Mux/2
  StateMap/1 -> Demux/1
  Mux/1 -> StateMap/1

== system suspention/DYN/CIntegrator/NthOrder1 ==
  u : Inport
  Demux : Demux  Outputs=[no no*N]
  Integrator : Integrator  InitialCondition=X0
  Mux : Mux  Inputs=[no no*N]
  StateMap : Selector  InputPortWidth=no*(1+N)  IndexOptions=Index vector (dialog)  Indices=stateMap  OutputSizes=1
  y : Outport
  wires:
  Mux/1 -> StateMap/1
  StateMap/1 -> Demux/1
  Integrator/1 -> Mux/2
  Demux/2 -> Integrator/1
  u/1 -> Mux/1
  Demux/1 -> y/1

== system suspention/DYN/CPIDControlLaw/D Term ==
  e : Inport
  Enable D Term : EnablePort  StatesWhenEnabling=reset  PropagateVarSize=During execution
  Derivative : Gain  Gain=D  SaturateOnIntegerOverflow=on  OutDataTypeStr=Inherit: Same as input  ParamDataTypeStr=Inherit: Same as input
  Sum1 : Sum  Inputs=|+-  SaturateOnIntegerOverflow=on  InputSameDT=on  OutDataTypeStr=Inherit: Same as first input
  TimeConstant : Gain  Gain=1/TAU  SaturateOnIntegerOverflow=on  OutDataTypeStr=Inherit: Same as input  ParamDataTypeStr=Inherit: Same as input
  xd : Integrator  InitialCondition=xd
  u_d : Outport
  wires:
  e/1 -> Sum1/1
  xd/1 -> Sum1/2
  TimeConstant/1 -> xd/1, Derivative/1
  Sum1/1 -> TimeConstant/1
  Derivative/1 -> u_d/1

== system suspention/DYN/CPIDControlLaw/I Term ==
  e : Inport
  Enable I Term : EnablePort  StatesWhenEnabling=reset  PropagateVarSize=During execution
  Integral : Gain  Gain=I  SaturateOnIntegerOverflow=on  OutDataTypeStr=Inherit: Same as input  ParamDataTypeStr=Inherit: Same as input
  xi : Integrator  InitialCondition=xi
  u_i : Outport
  wires:
  e/1 -> xi/1
  xi/1 -> Integral/1
  Integral/1 -> u_i/1

== system suspention/DYN/CResetIntegrator/1stOrder ==
  u : Inport
  new : Inport  Port=2
  reset : Inport  Port=3
  Gain : Gain  Gain=K  SaturateOnIntegerOverflow=on  OutDataTypeStr=Inherit: Same as input  ParamDataTypeStr=Inherit: Same as input
  IC : InitialCondition  Value=X0
  Integrator : Integrator  ExternalReset=rising  InitialConditionSource=external  InitialCondition=X0
  y : Outport
  wires:
  reset/1 -> Integrator/2
  IC/1 -> Integrator/3
  new/1 -> IC/1
  u/1 -> Integrator/1
  Integrator/1 -> Gain/1
  Gain/1 -> y/1

== system suspention/DYN/CResetIntegrator/1stOrder1 ==
  u : Inport
  new : Inport  Port=2
  reset : Inport  Port=3
  IC : InitialCondition  Value=X0
  Integrator : Integrator  ExternalReset=rising  InitialConditionSource=external  InitialCondition=X0
  y : Outport
  wires:
  Integrator/1 -> y/1
  u/1 -> Integrator/1
  new/1 -> IC/1
  IC/1 -> Integrator/3
  reset/1 -> Integrator/2

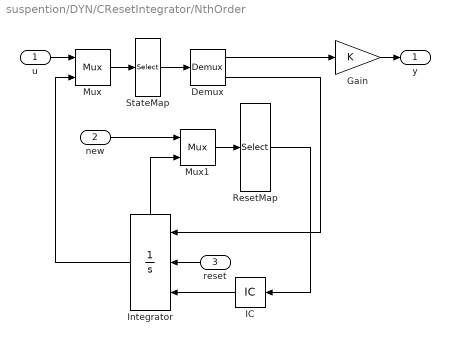
== system suspention/DYN/CResetIntegrator/NthOrder ==
  u : Inport
  new : Inport  Port=2
  reset : Inport  Port=3
  Demux : Demux  Outputs=[no no*N]
  Gain : Gain  Gain=K  SaturateOnIntegerOverflow=on  OutDataTypeStr=Inherit: Same as input  ParamDataTypeStr=Inherit: Same as input
  IC : InitialCondition  Value=X0
  Integrator : Integrator  ExternalReset=rising  InitialConditionSource=external  InitialCondition=X0  ShowStatePort=on
  Mux : Mux  Inputs=[no no*N]
  Mux1 : Mux  Inputs=[NR N]*no
  ResetMap : Selector  InputPortWidth=(NR+N)*no  IndexOptions=Index vector (dialog)  Indices=resetMap  OutputSizes=1
  StateMap : Selector  InputPortWidth=no*(1+N)  IndexOptions=Index vector (dialog)  Indices=stateMap  OutputSizes=1
  y : Outport
  wires:
  Demux/1 -> Gain/1
  u/1 -> Mux/1
  StateMap/1 -> Demux/1
  Mux/1 -> StateMap/1
  IC/1 -> Integrator/3
  Integrator/1 -> Mux/2
  reset/1 -> Integrator/2
  ResetMap/1 -> IC/1
  new/1 -> Mux1/1
  Mux1/1 -> ResetMap/1
  Integrator/State -> Mux1/2
  Gain/1 -> y/1
  Demux/2 -> Integrator/1

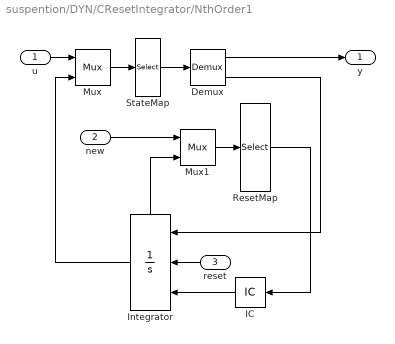
== system suspention/DYN/CResetIntegrator/NthOrder1 ==
  u : Inport
  new : Inport  Port=2
  reset : Inport  Port=3
  Demux : Demux  Outputs=[no no*N]
  IC : InitialCondition  Value=X0
  Integrator : Integrator  ExternalReset=rising  InitialConditionSource=external  InitialCondition=X0  ShowStatePort=on
  Mux : Mux  Inputs=[no no*N]
  Mux1 : Mux  Inputs=[NR N]*no
  ResetMap : Selector  InputPortWidth=(NR+N)*no  IndexOptions=Index vector (dialog)  Indices=resetMap  OutputSizes=1
  StateMap : Selector  InputPortWidth=no*(1+N)  IndexOptions=Index vector (dialog)  Indices=stateMap  OutputSizes=1
  y : Outport
  wires:
  Demux/2 -> Integrator/1
  Integrator/State -> Mux1/2
  Mux1/1 -> ResetMap/1
  new/1 -> Mux1/1
  ResetMap/1 -> IC/1
  reset/1 -> Integrator/2
  Integrator/1 -> Mux/2
  IC/1 -> Integrator/3
  Mux/1 -> StateMap/1
  StateMap/1 -> Demux/1
  u/1 -> Mux/1
  Demux/1 -> y/1

== system suspention/DYN/DIntegrator/1stOrder ==
  u : Inport  SampleTime=TS
  Gain : Gain  Gain=K  SaturateOnIntegerOverflow=on  OutDataTypeStr=Inherit: Same as input  ParamDataTypeStr=Inherit: Same as input
  Integrator : DiscreteIntegrator  InitialCondition=X0  SampleTime=TS  ICPrevOutput=DiscIntNeverNeededParam  ICPrevScaledInput=DiscIntNeverNeededParam
  y : Outport
  wires:
  u/1 -> Integrator/1
  Gain/1 -> y/1
  Integrator/1 -> Gain/1

== system suspention/DYN/DIntegrator/NthOrder ==
  u : Inport  SampleTime=TS
  Demux : Demux  Outputs=[no no*N]
  Gain : Gain  Gain=K  SaturateOnIntegerOverflow=on  OutDataTypeStr=Inherit: Same as input  ParamDataTypeStr=Inherit: Same as input
  Integrator : DiscreteIntegrator  InitialCondition=X0  SampleTime=TS  ICPrevOutput=DiscIntNeverNeededParam  ICPrevScaledInput=DiscIntNeverNeededParam
  Mux : Mux  Inputs=[no no*N]
  StateMap : Selector  InputPortWidth=no*(1+N)  IndexOptions=Index vector (dialog)  Indices=stateMap  OutputSizes=1
  y : Outport
  wires:
  Mux/1 -> StateMap/1
  StateMap/1 -> Demux/1
  Integrator/1 -> Mux/2
  Demux/2 -> Integrator/1
  u/1 -> Mux/1
  Demux/1 -> Gain/1
  Gain/1 -> y/1

== system suspention/DYN/DIntegrator/NthOrder1 ==
  u : Inport  SampleTime=TS
  Demux : Demux  Outputs=[no no*N]
  Integrator : DiscreteIntegrator  InitialCondition=X0  SampleTime=TS  ICPrevOutput=DiscIntNeverNeededParam  ICPrevScaledInput=DiscIntNeverNeededParam
  Mux : Mux  Inputs=[no no*N]
  StateMap : Selector  InputPortWidth=no*(1+N)  IndexOptions=Index vector (dialog)  Indices=stateMap  OutputSizes=1
  y : Outport
  wires:
  u/1 -> Mux/1
  Demux/2 -> Integrator/1
  Integrator/1 -> Mux/2
  StateMap/1 -> Demux/1
  Mux/1 -> StateMap/1
  Demux/1 -> y/1

== system suspention/DYN/DPIDControlLaw/D Term ==
  e : Inport
  Enable D Term : EnablePort  StatesWhenEnabling=reset  PropagateVarSize=During execution
  Derivative : Gain  Gain=D  SaturateOnIntegerOverflow=on  OutDataTypeStr=Inherit: Same as input  ParamDataTypeStr=Inherit: Same as input
  Sum1 : Sum  Inputs=-++  SaturateOnIntegerOverflow=on  InputSameDT=on  OutDataTypeStr=Inherit: Same as first input
  TimeConstant2 : Gain  Gain=1/(TAU+TS(1))  SaturateOnIntegerOverflow=on  OutDataTypeStr=Inherit: Same as input  ParamDataTypeStr=Inherit: Same as input
  TimeConstant3 : Gain  Gain=TAU  SaturateOnIntegerOverflow=on  OutDataTypeStr=Inherit: Same as input  ParamDataTypeStr=Inherit: Same as input
  ed : UnitDelay  SampleTime=TS  HasFrameUpgradeWarning=on
  xd : UnitDelay  InitialCondition=xd  SampleTime=TS  HasFrameUpgradeWarning=on
  u_d : Outport
  wires:
  TimeConstant2/1 -> Derivative/1, xd/1
  Derivative/1 -> u_d/1
  xd/1 -> TimeConstant3/1
  Sum1/1 -> TimeConstant2/1
  TimeConstant3/1 -> Sum1/3
  ed/1 -> Sum1/1
  e/1 -> Sum1/2, ed/1

== system suspention/DYN/DPIDControlLaw/I Term ==
  e : Inport
  Enable I Term : EnablePort  StatesWhenEnabling=reset  PropagateVarSize=During execution
  Integral : Gain  Gain=I  SaturateOnIntegerOverflow=on  OutDataTypeStr=Inherit: Same as input  ParamDataTypeStr=Inherit: Same as input
  Sum2 : Sum  SaturateOnIntegerOverflow=on  InputSameDT=on  OutDataTypeStr=Inherit: Same as first input
  TimeConstant1 : Gain  Gain=TS(1)  SaturateOnIntegerOverflow=on  OutDataTypeStr=Inherit: Same as input  ParamDataTypeStr=Inherit: Same as input
  xi : UnitDelay  InitialCondition=xi  SampleTime=TS  HasFrameUpgradeWarning=on
  u_i : Outport
  wires:
  e/1 -> TimeConstant1/1
  TimeConstant1/1 -> Sum2/1
  xi/1 -> Sum2/2
  Sum2/1 -> xi/1, Integral/1
  Integral/1 -> u_i/1

== system suspention/DYN/DResetIntegrator/1stOrder ==
  u : Inport  SampleTime=TS
  new : Inport  Port=2  SampleTime=TS
  reset : Inport  Port=3  SampleTime=TS
  Gain : Gain  Gain=K  SaturateOnIntegerOverflow=on  OutDataTypeStr=Inherit: Same as input  ParamDataTypeStr=Inherit: Same as input
  IC : InitialCondition  Value=X0
  Integrator : DiscreteIntegrator  ExternalReset=rising  InitialConditionSource=external  InitialCondition=X0  SampleTime=TS  ICPrevOutput=DiscIntNeverNeededParam  ICPrevScaledInput=DiscIntNeverNeededParam
  y : Outport
  wires:
  IC/1 -> Integrator/3
  reset/1 -> Integrator/2
  new/1 -> IC/1
  u/1 -> Integrator/1
  Gain/1 -> y/1
  Integrator/1 -> Gain/1

== system suspention/DYN/DResetIntegrator/1stOrder1 ==
  u : Inport  SampleTime=TS
  new : Inport  Port=2  SampleTime=TS
  reset : Inport  Port=3  SampleTime=TS
  IC : InitialCondition  Value=X0
  Integrator : DiscreteIntegrator  ExternalReset=rising  InitialConditionSource=external  InitialCondition=X0  SampleTime=TS  ICPrevOutput=DiscIntNeverNeededParam  ICPrevScaledInput=DiscIntNeverNeededParam
  y : Outport
  wires:
  u/1 -> Integrator/1
  new/1 -> IC/1
  reset/1 -> Integrator/2
  IC/1 -> Integrator/3
  Integrator/1 -> y/1

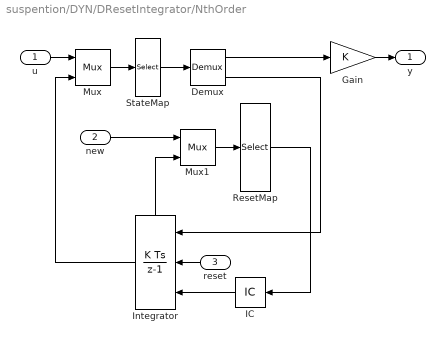
== system suspention/DYN/DResetIntegrator/NthOrder ==
  u : Inport  SampleTime=TS
  new : Inport  Port=2  SampleTime=TS
  reset : Inport  Port=3  SampleTime=TS
  Demux : Demux  Outputs=[no no*N]
  Gain : Gain  Gain=K  SaturateOnIntegerOverflow=on  OutDataTypeStr=Inherit: Same as input  ParamDataTypeStr=Inherit: Same as input
  IC : InitialCondition  Value=X0
  Integrator : DiscreteIntegrator  ExternalReset=rising  InitialConditionSource=external  InitialCondition=X0  SampleTime=TS  ShowStatePort=on  ICPrevOutput=DiscIntNeverNeededParam  ICPrevScaledInput=DiscIntNeverNeededParam
  Mux : Mux  Inputs=[no no*N]
  Mux1 : Mux  Inputs=[NR N]*no
  ResetMap : Selector  InputPortWidth=(NR+N)*no  IndexOptions=Index vector (dialog)  Indices=resetMap  OutputSizes=1
  StateMap : Selector  InputPortWidth=no*(1+N)  IndexOptions=Index vector (dialog)  Indices=stateMap  OutputSizes=1
  y : Outport
  wires:
  Demux/1 -> Gain/1
  u/1 -> Mux/1
  StateMap/1 -> Demux/1
  Mux/1 -> StateMap/1
  IC/1 -> Integrator/3
  Integrator/1 -> Mux/2
  reset/1 -> Integrator/2
  ResetMap/1 -> IC/1
  new/1 -> Mux1/1
  Mux1/1 -> ResetMap/1
  Integrator/State -> Mux1/2
  Gain/1 -> y/1
  Demux/2 -> Integrator/1

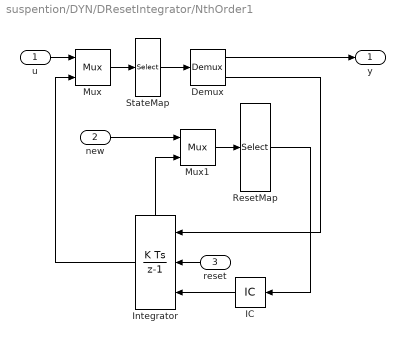
== system suspention/DYN/DResetIntegrator/NthOrder1 ==
  u : Inport  SampleTime=TS
  new : Inport  Port=2  SampleTime=TS
  reset : Inport  Port=3  SampleTime=TS
  Demux : Demux  Outputs=[no no*N]
  IC : InitialCondition  Value=X0
  Integrator : DiscreteIntegrator  ExternalReset=rising  InitialConditionSource=external  InitialCondition=X0  SampleTime=TS  ShowStatePort=on  ICPrevOutput=DiscIntNeverNeededParam  ICPrevScaledInput=DiscIntNeverNeededParam
  Mux : Mux  Inputs=[no no*N]
  Mux1 : Mux  Inputs=[NR N]*no
  ResetMap : Selector  InputPortWidth=(NR+N)*no  IndexOptions=Index vector (dialog)  Indices=resetMap  OutputSizes=1
  StateMap : Selector  InputPortWidth=no*(1+N)  IndexOptions=Index vector (dialog)  Indices=stateMap  OutputSizes=1
  y : Outport
  wires:
  Demux/2 -> Integrator/1
  Integrator/State -> Mux1/2
  Mux1/1 -> ResetMap/1
  new/1 -> Mux1/1
  ResetMap/1 -> IC/1
  reset/1 -> Integrator/2
  Integrator/1 -> Mux/2
  IC/1 -> Integrator/3
  Mux/1 -> StateMap/1
  StateMap/1 -> Demux/1
  u/1 -> Mux/1
  Demux/1 -> y/1
